simulink model "sampleModel1684_sub_sub"  (R2023a)
settings: Solver=VariableStepAuto  StartTime=0.0  StopTime=10.0  RelTol=1e-3
libraries: hdlsllib x5, simulink x3
settings Model: Creator=user1  LastModifiedBy=user1
settings OptimizationCC: BlockReduction=off  ConditionallyExecuteInputs=off

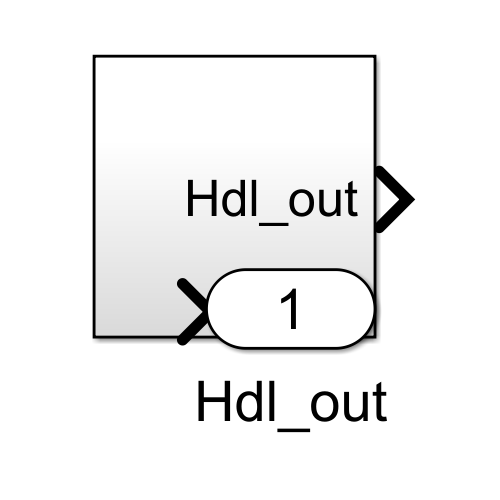
[thumbnail: Simulink's stored preview of the top-level diagram]
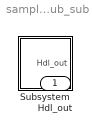
== system sampleModel1684_sub_sub ==
  Subsystem : Subsystem
  Hdl_out : Outport  OutDataTypeStr=uint8

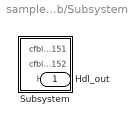
== system sampleModel1684_sub_sub/Subsystem ==
  Subsystem : Subsystem
  Hdl_out : Outport  OutDataTypeStr=uint8

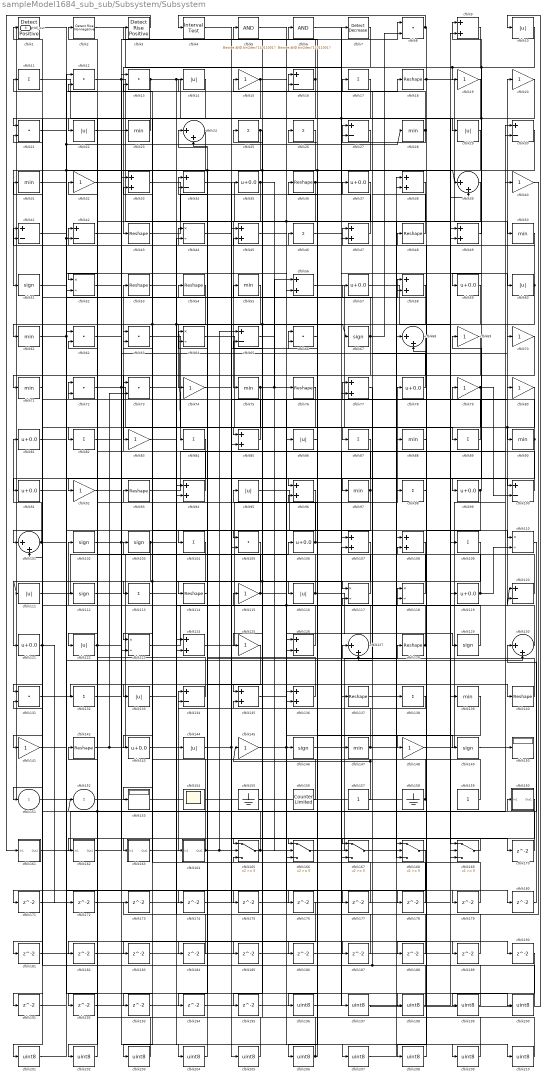
== system sampleModel1684_sub_sub/Subsystem/Subsystem ==
  cfblk1 : hdlsllib/Logic and Bit Operations/Detect Rise Positive  vinit=0  OutDataTypeStr=uint8
  cfblk{10,14,22,29,60,86,95,111,116,122,133,144} (12 alike) : Abs  OutDataTypeStr=uint8  SaturateOnIntegerOverflow=off
  cfblk{16,27,30,34,41..42,65,100,120,134} (10 alike) : Sum  Inputs=+-  OutDataTypeStr=uint8
  cfblk{24,39,68,101,127,130} (6 alike) : Sum  Inputs=|++  OutDataTypeStr=uint8
  cfblk{51,67,102..103,112,129,146,149} (8 alike) : Signum
  cfblk{11,17,25..26,46,82,84,87,89,98,104,109,113,132,138} (15 alike) : Sum  Inputs=+  OutDataTypeStr=uint8
  cfblk{8,12..13,21,62..63,66,72..73,105,131} (11 alike) : DotProduct  OutDataTypeStr=uint8
  cfblk{35,37,57,59,78,81,91,99,106,119,121,143} (12 alike) : Bias  Bias=0.0  SaturateOnIntegerOverflow=off
  cfblk{9,33,38,45,47,49,56,58,77,85,94,96,107..108,124,126,135..136} (18 alike) : Sum  OutDataTypeStr=uint8
  cfblk{44,52,64,110,117..118,123} (7 alike) : Product  Inputs=*/  OutDataTypeStr=uint8  RndMeth=Zero  SaturateOnIntegerOverflow=on
  cfblk{18,36,43,48,53..54,76,93,114,128,137,140,142} (13 alike) : Reshape
  cfblk{15,19..20,32,40,69..70,74,79..80,83,92,115,125,141,145,148} (17 alike) : Gain  OutDataTypeStr=uint8
  cfblk{23,28,31,50,55,61,71,75,88,90,97,139,147} (13 alike) : MinMax  OutDataTypeStr=uint8
  cfblk150 : Display
  cfblk153 : Display
  cfblk154 : Scope
      settings: Floating=on
  cfblk155 : Ground
  cfblk156 : hdlsllib/Sources/Counter Limited  uplimit=7  tsamp=-1
  cfblk157 : Constant  OutDataTypeStr=uint8  SampleTime=-1
  cfblk158 : Ground
  cfblk159 : Constant  OutDataTypeStr=uint8  SampleTime=-1
  cfblk160 : Subsystem
      settings: LibrarySourceBlock=|
      | hdlsllib/Ports &
      | Subsystems/Subsystem
  cfblk161 : Subsystem
      settings: LibrarySourceBlock=|
      | hdlsllib/Ports &
      | Subsystems/Subsystem
  cfblk162 : Subsystem
      settings: LibrarySourceBlock=|
      | hdlsllib/Ports &
      | Subsystems/Subsystem
  cfblk163 : Subsystem
      settings: LibrarySourceBlock=|
      | hdlsllib/Ports &
      | Subsystems/Subsystem
  cfblk164 : Subsystem
      settings: LibrarySourceBlock=|
      | hdlsllib/Ports &
      | Subsystems/Subsystem
  cfblk{165..169} (5 alike) : Switch  OutDataTypeStr=uint8  SaturateOnIntegerOverflow=off  InputSameDT=off
  cfblk{170..195} (26 alike) : Delay  SampleTime=1
  cfblk{196..210} (15 alike) : DataTypeConversion  OutDataTypeStr=uint8  SaturateOnIntegerOverflow=off  RndMeth=Floor
  cfblk2 : hdlsllib/Logic and Bit Operations/Detect Rise Nonnegative  vinit=0  OutDataTypeStr=uint8
  cfblk3 : hdlsllib/Logic and Bit Operations/Detect Rise Positive  vinit=0  OutDataTypeStr=uint8
  cfblk4 : hdlsllib/Logic and Bit Operations/Interval Test  IntervalClosedRight=on  uplimit=0.5  IntervalClosedLeft=on  lowlimit=-0.5  OutDataTypeStr=uint8
  cfblk5 : simulink/Logic and Bit Operations/Bitwise Operator  logicop=AND  UseBitMask=on  BitMask=bin2dec('11011001')  BitMaskRealWorld=Stored Integer
      settings: LibrarySourceBlock=|
      | hdlsllib/Logic and Bit
      | Operations/Bitwise
      | Operator
  cfblk6 : simulink/Logic and Bit Operations/Bitwise Operator  logicop=AND  UseBitMask=on  BitMask=bin2dec('11011001')  BitMaskRealWorld=Stored Integer
      settings: LibrarySourceBlock=|
      | hdlsllib/Logic and Bit
      | Operations/Bitwise
      | Operator
  cfblk7 : simulink/Logic and Bit Operations/Detect Decrease  vinit=0.0  OutDataTypeStr=uint8
      settings: LibrarySourceBlock=|
      | hdlsllib/Logic and Bit
      | Operations/Detect
      | Decrease
  cfblk151 : Outport  OutDataTypeStr=uint8  VectorParamsAs1DForOutWhenUnconnected=off
  cfblk152 : Outport  Port=2  OutDataTypeStr=uint8  VectorParamsAs1DForOutWhenUnconnected=off
  Hdl_out : Outport  Port=3  OutDataTypeStr=uint8
  wires:
  cfblk210/1 -> cfblk96/2
  cfblk5/1 -> cfblk210/1
  cfblk209/1 -> cfblk5/1
  cfblk44/1 -> cfblk209/1
  cfblk208/1 -> cfblk108/2
  cfblk207/1 -> cfblk108/1
  cfblk113/1 -> cfblk207/1
  cfblk206/1 -> cfblk142/1, cfblk26/1
  cfblk205/1 -> cfblk24/2
  cfblk194/1 -> cfblk205/1
  cfblk204/1 -> cfblk24/1
  cfblk82/1 -> cfblk204/1
  cfblk203/1 -> cfblk12/2, cfblk152/1
  cfblk202/1 -> cfblk62/2
  cfblk176/1 -> cfblk202/1
  cfblk201/1 -> cfblk62/1
  cfblk71/1 -> cfblk201/1
  cfblk200/1 -> cfblk131/2, cfblk57/1
  cfblk199/1 -> cfblk1/1
  cfblk190/1 -> cfblk199/1
  cfblk198/1 -> cfblk95/1
  cfblk1/1 -> cfblk198/1
  cfblk197/1 -> cfblk10/1
  cfblk6/1 -> cfblk197/1
  cfblk196/1 -> cfblk6/1
  cfblk139/1 -> cfblk196/1
  cfblk195/1 -> cfblk165/3
  cfblk125/1 -> cfblk194/1
  cfblk193/1 -> cfblk169/3
  cfblk192/1 -> cfblk167/2
  cfblk191/1 -> cfblk12/1
  cfblk83/1 -> cfblk190/1
  cfblk189/1 -> cfblk169/2
  cfblk52/1 -> cfblk189/1
  cfblk188/1 -> cfblk127/2
  cfblk187/1 -> cfblk34/2
  cfblk186/1 -> cfblk167/3
  cfblk185/1 -> cfblk135/2
  cfblk184/1 -> cfblk124/1
  cfblk183/1 -> cfblk38/2
  cfblk182/1 -> cfblk49/1
  cfblk160/1(Out1) -> cfblk182/1
  cfblk181/1 -> cfblk39/2
  cfblk168/1 -> cfblk181/1
  cfblk180/1 -> cfblk130/1
  cfblk46/1 -> cfblk180/1
  cfblk179/1 -> cfblk126/1
  cfblk112/1 -> cfblk179/1
  cfblk178/1 -> cfblk94/1
  cfblk132/1 -> cfblk178/1
  cfblk177/1 -> cfblk63/2
  cfblk141/1 -> cfblk177/1
  cfblk133/1 -> cfblk176/1
  cfblk175/1 -> cfblk107/2
  cfblk174/1 -> cfblk68/1
  cfblk96/1 -> cfblk174/1
  cfblk173/1 -> cfblk136/1
  cfblk40/1 -> cfblk173/1
  cfblk172/1 -> cfblk165/2
  cfblk171/1 -> cfblk9/2
  cfblk170/1 -> cfblk13/1
  cfblk158/1 -> cfblk33/2, Hdl_out/1
  cfblk117/1 -> cfblk2/1
  cfblk41/1 -> cfblk112/1
  cfblk11/1 -> cfblk107/1
  cfblk13/1 -> cfblk94/2, cfblk139/1, cfblk122/1
  cfblk155/1 -> cfblk115/1
  cfblk85/1 -> cfblk73/1
  cfblk147/1 -> cfblk120/2, cfblk25/1
  cfblk118/1 -> cfblk46/1
  cfblk70/1 -> cfblk125/1
  cfblk30/1 -> cfblk113/1
  cfblk134/1 -> cfblk72/2
  cfblk73/1 -> cfblk116/1
  cfblk15/1 -> cfblk29/1, cfblk193/1
  cfblk7/1 -> cfblk77/2
  cfblk81/1 -> cfblk130/2
  cfblk165/1 -> cfblk31/1, cfblk98/1
  cfblk16/1 -> cfblk105/2, cfblk3/1
  cfblk29/1 -> cfblk104/1, cfblk191/1
  cfblk109/1 -> cfblk111/1, cfblk175/1
  cfblk48/1 -> cfblk17/1
  cfblk164/1(Out1) -> cfblk77/1, cfblk65/1, cfblk93/1
  cfblk21/1 -> cfblk42/2, cfblk56/2
  cfblk4/1 -> cfblk117/1
  cfblk60/1 -> cfblk45/2, cfblk162/1(In1)
  cfblk137/1 -> cfblk38/1
  cfblk116/1 -> cfblk168/2, cfblk64/2
  cfblk26/1 -> cfblk105/1, cfblk52/2
  cfblk2/1 -> cfblk147/1
  cfblk50/1 -> cfblk41/2
  cfblk108/1 -> cfblk206/1
  cfblk32/1 -> cfblk16/2
  cfblk51/1 -> cfblk132/1
  cfblk140/1 -> cfblk54/1
  cfblk14/1 -> cfblk153/1
  cfblk95/1 -> cfblk137/1
  cfblk167/1 -> cfblk79/1
  cfblk66/1 -> cfblk16/1
  cfblk90/1 -> cfblk41/1, cfblk101/2
  cfblk149/1 -> cfblk150/1
  cfblk36/1 -> cfblk60/1, cfblk195/1
  cfblk33/1 -> cfblk138/1
  cfblk74/1 -> cfblk35/1
  cfblk86/1 -> cfblk66/1
  cfblk38/1 -> cfblk165/1
  cfblk111/1 -> cfblk44/2
  cfblk23/1 -> cfblk21/1
  cfblk78/1 -> cfblk47/1
  cfblk76/1 -> cfblk85/1
  cfblk88/1 -> cfblk58/2
  cfblk72/1 -> cfblk168/3, cfblk184/1
  cfblk59/1 -> cfblk74/1
  cfblk68/1 -> cfblk71/1
  cfblk115/1 -> cfblk86/1, cfblk64/1
  cfblk34/1 -> cfblk169/1
  cfblk54/1 -> cfblk123/2
  cfblk169/1 -> cfblk167/1
  cfblk162/1(Out1) -> cfblk70/1
  cfblk121/1 -> cfblk171/1, cfblk172/1
  cfblk47/1 -> cfblk37/1
  cfblk99/1 -> cfblk148/1, cfblk69/1
  cfblk114/1 -> cfblk44/1
  cfblk166/1 -> cfblk118/2
  cfblk102/1 -> cfblk33/1, cfblk186/1
  cfblk43/1 -> cfblk7/1
  cfblk146/1 -> cfblk128/1
  cfblk107/1 -> cfblk126/2
  cfblk49/1 -> cfblk9/1
  cfblk126/1 -> cfblk63/1
  cfblk28/1 -> cfblk15/1, cfblk27/2
  cfblk91/1 -> cfblk58/1
  cfblk106/1 -> cfblk72/1, cfblk88/1
  cfblk92/1 -> cfblk23/1
  cfblk3/1 -> cfblk161/1(In1)
  cfblk103/1 -> cfblk164/1(In1), cfblk131/1
  cfblk22/1 -> cfblk168/1
  cfblk63/1 -> cfblk119/1
  cfblk120/1 -> cfblk27/1
  cfblk42/1 -> cfblk97/1
  cfblk135/1 -> cfblk120/1, cfblk80/1
  cfblk93/1 -> cfblk30/2
  cfblk124/1 -> cfblk78/1
  cfblk69/1 -> cfblk83/1
  cfblk119/1 -> cfblk13/2, cfblk110/2
  cfblk100/1 -> cfblk36/1
  cfblk62/1 -> cfblk200/1
  cfblk145/1 -> cfblk149/1
  cfblk105/1 -> cfblk121/1
  cfblk75/1 -> cfblk129/1, cfblk56/1, cfblk91/1
  cfblk39/1 -> cfblk136/2, cfblk52/1
  cfblk84/1 -> cfblk92/1
  cfblk123/1 -> cfblk45/1
  cfblk27/1 -> cfblk96/1, cfblk141/1
  cfblk45/1 -> cfblk146/1, cfblk187/1
  cfblk122/1 -> cfblk42/1, cfblk8/1
  cfblk89/1 -> cfblk55/1
  cfblk128/1 -> cfblk68/2, cfblk117/2
  cfblk87/1 -> cfblk166/1
  cfblk138/1 -> cfblk134/2
  cfblk19/1 -> cfblk61/1
  cfblk143/1 -> cfblk118/1
  cfblk129/1 -> cfblk102/1
  cfblk8/1 -> cfblk4/1, cfblk188/1
  cfblk17/1 -> cfblk151/1, cfblk47/2
  cfblk98/1 -> cfblk48/1
  cfblk144/1 -> cfblk66/2, cfblk170/1
  cfblk61/1 -> cfblk28/1, cfblk18/1, cfblk100/1
  cfblk53/1 -> cfblk144/1, cfblk67/1
  cfblk67/1 -> cfblk123/1, cfblk21/2, cfblk8/2
  cfblk79/1 -> cfblk82/1, cfblk100/2
  cfblk35/1 -> cfblk114/1, cfblk166/2
  cfblk31/1 -> cfblk39/1, cfblk14/1
  cfblk57/1 -> cfblk109/1
  cfblk20/1 -> cfblk59/1, cfblk85/2
  cfblk37/1 -> cfblk75/1
  cfblk163/1(Out1) -> cfblk134/1
  cfblk9/1 -> cfblk43/1
  cfblk101/1 -> cfblk81/1, cfblk110/1
  cfblk136/1 -> cfblk34/1
  cfblk161/1(Out1) -> cfblk40/1
  cfblk80/1 -> cfblk90/1, cfblk124/2
  cfblk156/1 -> cfblk103/1
  cfblk56/1 -> cfblk89/1
  cfblk97/1 -> cfblk32/1, cfblk183/1
  cfblk110/1 -> cfblk160/1(In1)
  cfblk157/1 -> cfblk145/1, cfblk65/2
  cfblk94/1 -> cfblk53/1
  cfblk58/1 -> cfblk84/1, cfblk185/1
  cfblk104/1 -> cfblk143/1, cfblk192/1
  cfblk148/1 -> cfblk30/1
  cfblk77/1 -> cfblk127/1
  cfblk127/1 -> cfblk11/1
  cfblk10/1 -> cfblk19/1, cfblk166/3, cfblk99/1
  cfblk24/1 -> cfblk203/1
  cfblk64/1 -> cfblk87/1
  cfblk12/1 -> cfblk49/2, cfblk140/1
  cfblk65/1 -> cfblk76/1
  cfblk55/1 -> cfblk163/1(In1), cfblk101/1
  cfblk18/1 -> cfblk50/1, cfblk208/1
  cfblk159/1 -> cfblk22/1
  cfblk131/1 -> cfblk133/1
  cfblk130/1 -> cfblk20/1
  cfblk142/1 -> cfblk106/1, cfblk73/2
  cfblk25/1 -> cfblk51/1, cfblk135/1

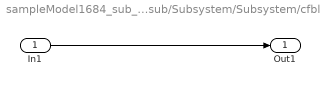
== system sampleModel1684_sub_sub/Subsystem/Subsystem/cfblk160 ==
  In1 : Inport
  Out1 : Outport
  wires:
  In1/1 -> Out1/1

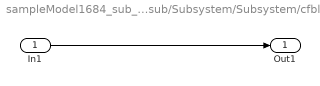
== system sampleModel1684_sub_sub/Subsystem/Subsystem/cfblk161 ==
  In1 : Inport
  Out1 : Outport
  wires:
  In1/1 -> Out1/1

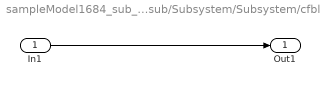
== system sampleModel1684_sub_sub/Subsystem/Subsystem/cfblk162 ==
  In1 : Inport
  Out1 : Outport
  wires:
  In1/1 -> Out1/1

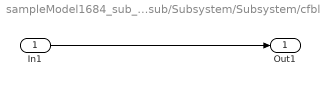
== system sampleModel1684_sub_sub/Subsystem/Subsystem/cfblk163 ==
  In1 : Inport
  Out1 : Outport
  wires:
  In1/1 -> Out1/1

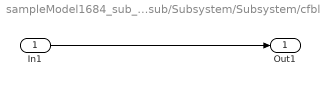
== system sampleModel1684_sub_sub/Subsystem/Subsystem/cfblk164 ==
  In1 : Inport
  Out1 : Outport
  wires:
  In1/1 -> Out1/1
